simulink model "satellite_11_scenario_1"  (R2021a)
settings: Solver=VariableStepAuto  StartTime=0.0  StopTime=10.0  RelTol=1e-3
libraries: fuzblock x1
settings Model: Creator=User  LastModifiedBy=User

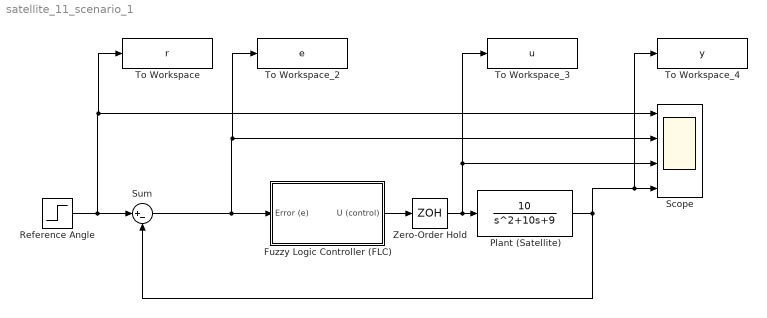
== system satellite_11_scenario_1 ==
  Fuzzy Logic Controller (FLC) : Subsystem
  Plant (Satellite) : TransferFcn  Numerator=[10]  Denominator=[1 10 9]
  Reference Angle : Step  After=50  SampleTime=0
  "Scope " : Scope  NumInputPorts=4
  Sum : Sum  Inputs=|+-
  "To Workspace " : ToWorkspace  VariableName=r  SaveFormat=Timeseries  SampleTime=-1
  To Workspace_2 : ToWorkspace  VariableName=e  SaveFormat=Timeseries  SampleTime=-1
  To Workspace_3 : ToWorkspace  VariableName=u  SaveFormat=Timeseries  SampleTime=-1
  To Workspace_4 : ToWorkspace  VariableName=y  SaveFormat=Timeseries  SampleTime=-1
  Zero-Order Hold : ZeroOrderHold  SampleTime=-1
  wires:
  Reference Angle/1 -> "To Workspace "/1, "Scope "/1, Sum/1
  Plant (Satellite)/1 -> To Workspace_4/1, "Scope "/4, Sum/2
  Sum/1 -> To Workspace_2/1, "Scope "/2, Fuzzy Logic Controller (FLC)/1(Error (e))
  Fuzzy Logic Controller (FLC)/1("\tU (control)") -> Zero-Order Hold/1
  Zero-Order Hold/1 -> To Workspace_3/1, "Scope "/3, Plant (Satellite)/1

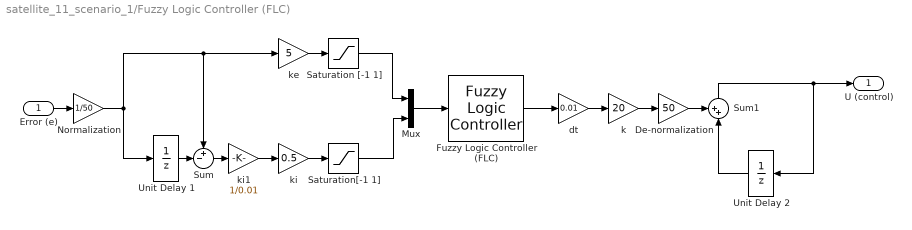
== system satellite_11_scenario_1/Fuzzy Logic Controller (FLC) ==
  Error (e) : Inport
  De-normalization : Gain  Gain=50
  Fuzzy Logic Controller (FLC) : fuzblock/Fuzzy Logic  Controller  FIS='fis_satellite.fis'  OutputSampleNumber=101  DataType=double  FuzzifiedInputs=off  RuleFiringStrengths=off  RuleOutputs=off  AggregatedOutputs=off  SimulateUsing=Interpreted execution  OutOfRangeInputValueMessage=warning  NoRuleFiredMessage=warning  EmptyOutputFuzzySetMessage=warning
  Mux : Mux  Inputs=2
  Normalization : Gain  Gain=1/50
  Saturation [-1 1] : Saturate  UpperLimit=1  LowerLimit=-1
  "Saturation[-1 1] " : Saturate  UpperLimit=1  LowerLimit=-1
  Sum : Sum  Inputs=+-|
  Sum1 : Sum  Inputs=++|
  Unit Delay 1 : UnitDelay  SampleTime=0.01  HasFrameUpgradeWarning=on
  Unit Delay 2 : UnitDelay  SampleTime=0.01  HasFrameUpgradeWarning=on
  dt : Gain  Gain=0.01
  k : Gain  Gain=20
  ke : Gain  Gain=5
  ki : Gain  Gain=0.5
  ki1 : Gain  Gain=1/0.01
  "\tU (control)" : Outport
  wires:
  Error (e)/1 -> Normalization/1
  Fuzzy Logic Controller (FLC)/1 -> dt/1
  Mux/1 -> Fuzzy Logic Controller (FLC)/1
  ki1/1 -> ki/1
  ke/1 -> Saturation [-1 1]/1
  Normalization/1 -> Unit Delay 1/1, Sum/1, ke/1
  Saturation [-1 1]/1 -> Mux/1
  "Saturation[-1 1] "/1 -> Mux/2
  Unit Delay 1/1 -> Sum/2
  Sum/1 -> ki1/1
  De-normalization/1 -> Sum1/1
  Unit Delay 2/1 -> Sum1/2
  ki/1 -> "Saturation[-1 1] "/1
  dt/1 -> k/1
  k/1 -> De-normalization/1
  Sum1/1 -> Unit Delay 2/1, "\tU (control)"/1
